simulink model "rule_DJ"  (R2021a)
settings: Solver=FixedStepAuto  StartTime=0.0  StopTime=8.9  FixedStep=1/30  RelTol=1e-3
values from neighbouring files (symbols this model uses):
  y = zeros(10,4)    [simulate.m]
libraries: simulink x17
(part 2 of 3)

== matlab function rule_DJ/EnabledSubsystem/EnabledSubsystem/changeright ==
  data: Egolane input; initial_lane input; Ego input; y1 output; y_line input; maxt_changeline output; staticinfo input; cmplt_change output
function [y1,maxt_changeline,cmplt_change] = fcn(Egolane,initial_lane,Ego,y_line,staticinfo)
%%参数注释
%{
sEgo = 0;                  %自车纵坐标（始终为零）(m)
dEgo = Ego(2);             %自车横坐标(m)
vxEgo = Ego(3);            %自车纵向速度(m/s)
vyEgo = Ego(4);            %自车横向速度(m/s)
phiEgo = Ego(5);           %自车航向角（相对路径切向夹角，逆时针为正） (rad)
laneEgo = Ego(6);          %自车所在车道
wEgo = Ego(7);             %自车横向宽度(m)
aEgo = Ego(8);             %自车质心到最前端的距离(m)
bEgo = Ego(9);             %自车质心到最前端的距离(m)
sTgt_ot = Tgt_ot(1);       %超车目标纵坐标(m)
dTgt_ot = Tgt_ot(2);       %超车目标横坐标(m)
vxTgt_ot = Tgt_ot(3);      %超车目标纵向速度(m/s)
vyTgt_ot = Tgt_ot(4);      %超车目标横向速度(m/s)
sTgt_f = Tgt_f(1);         %前车纵坐标(m)
dTgt_f = Tgt_f(2);         %前车横坐标(m)
vxTgt_f = Tgt_f(3);        %前车纵向速度(m/s)
vyTgt_f = Tgt_f(4);        %前车横向速度(m/s)
sTgt_lf = Tgt_lf(1);       %左前车纵坐标(m)
dTgt_lf = Tgt_lf(2);       %左前车横坐标(m)
vxTgt_lf = Tgt_lf(3);      %左前车纵向速度(m/s)
vyTgt_lf = Tgt_lf(4);      %左前车横向速度(m/s)
Tgt_lr, Tgt_rf, Tgt_rr与左前车类似，分别表示相对自车的左后车辆，右前车辆以及右后车辆
dlaneline =[dlaneline-1,dlaneline-2,……]
%同向车道内车道线横向坐标集，最靠近道路中心线的一侧为-1，往外依次递减
TTCx_f = Threshold_para(1);             %纵向安全距离
TTCx_lr = Threshold_para(2);            %超车道后方安全距离
TTCx_lf = Threshold_para(3);            %超车道前方安全距离
t_chngln = Threshold_para(4);           %换道持续最大时间
overtake_deltav = Threshold_para(5);    %超车速度差
sf_dist_return = Threshold_para(6);     %返回原车道与后方车辆的安全，由于超车时自车速度应大于被超车辆
TTCx_rf = Threshold_para(7);            %原车道前方安全距离
%}
%%

%参数需求
Egox = Ego.EgoX;
Egoy = Ego.EgoY;                    %自车y坐标(m)
Egovx = Ego.EgoVx;
Egovy = Ego.EgoVy;
Egol = Ego.Length;
Egow = Ego.Width;
Egotheta = Ego.EgoTheta;
laneEgo = Egolane;          %自车所在车道
maxt_changeline = staticinfo(6);


%计算向左换道所用时间
lf_Ego = Egoy + 0.5 * Egol * sin(Egotheta) - 0.5 * Egow * cos(Egotheta); %左前角车辆横坐标
rf_Ego = Egoy + 0.5 * Egol * sin(Egotheta) + 0.5 * Egow * cos(Egotheta); %右前角车辆横坐标
lr_Ego = Egoy - 0.5 * Egol * sin(Egotheta) - 0.5 * Egow * cos(Egotheta); %左前角车辆横坐标
rr_Ego = Egoy - 0.5 * Egol * sin(Egotheta) + 0.5 * Egow * cos(Egotheta); %右后角车辆横坐标
if Egovx > 0 && Egovy > 0
    changeleft = 1;
    Egoxf_line = polyval(y_line(initial_lane,:),Egox+0.5*Egol*cos(Egotheta));
    changeright = sign((rf_Ego-Egoxf_line) * (lr_Ego-Egoxf_line));
elseif Egovx > 0 && Egovy < 0
    Egoxf_line = polyval(y_line(initial_lane+1,:),Egox+0.5*Egol*cos(Egotheta));
    changeleft = sign((lf_Ego-Egoxf_line) * (rr_Ego-Egoxf_line));
    changeright = 1;
elseif Egovx < 0 && Egovy > 0
    Egoxf_line = polyval(y_line(initial_lane,:),Egox+0.5*Egol*cos(Egotheta));
    changeleft = sign((lf_Ego-Egoxf_line) * (rr_Ego-Egoxf_line));
    changeright = 1;
else
    changeleft = 1;
    Egoxf_line = polyval(y_line(initial_lane+1,:),Egox+0.5*Egol*cos(Egotheta));
    changeright = sign((rf_Ego-Egoxf_line) * (lr_Ego-Egoxf_line));
end

if changeright <= 0
    y1 = true;       %y1为true的时间即为换道时间，该时间不得超过10s
else
    y1 = false;
end

if laneEgo == initial_lane && changeleft > 0 && changeright > 0
    cmplt_change = 1;
elseif laneEgo ~= initial_lane && changeleft > 0 && changeright > 0
    cmplt_change = 2;
elseif laneEgo ~= initial_lane && changeright <= 0
    cmplt_change = 3;
else
    cmplt_change = 0;
end

end

== matlab function rule_DJ/trigger_rule78 ==
  data: y_line input; y output; Egolaneid input
function y = fcn(y_line,Egolaneid)
%%

%参数需求
lane_type = Egolaneid;

%高速主路限速触发条件判断
if lane_type ~= 1 && lane_type ~= size(y_line,1)-1        %自车所属车道类型为主干道则条件有效
    y = 1;
else
    y = 0;
end

== matlab function rule_DJ/EnabledSubsystem/EnabledSubsystem/distance/zoning ==
  data: Ego input; Tgt_f output; Tgt input; y_line input; Tgt_b output; Tgt_lf output; Tgt_lr output; Tgt_rf output; Tgt_rr output; Egolane output
function [Tgt_f,Tgt_b,Tgt_lf,Tgt_lr,Tgt_rf,Tgt_rr,Egolane] = fcn(Ego,Tgt,y_line)
%{
根据HighD数据集提供的信息，通过确定自车所在的位置，以及他车的坐标，判断他车相对于自车的方位
%}
Egox = Ego.EgoX;
Egoy = Ego.EgoY;
Egovx = Ego.EgoVx;
Tgtx = Tgt.TgtX;
Tgty = Tgt.TgtY;
Tgtvx = Tgt.TgtVx;
Tgtl = Tgt.Length;
Tgtw = Tgt.Width;

%%判断自车所在的车道
for i = 1:size(y_line,1)
    if Egoy >= polyval(y_line(i,:),Egox);
        Egolane = i-1;
        break
    else
        Egolane = i;
    end
end

%%对周围的他车进行方位分割
if Egolane<size(y_line,1)/2  %说明自车在地图中为向右行驶（下方）车辆
    Flag1 = Tgtx > Egox;      %他车位于自车之前
    Flag2 = Tgtx <= Egox;     %他车位于自车之后
    if Egolane == 1                                   %自车位于车道1
        Flag3 = (Tgty>=polyval(y_line(2,:),Tgtx) & Tgty<polyval(y_line(1,:),Tgtx));      %同车道他车
        Flag5 = (Tgty>=polyval(y_line(3,:),Tgtx) & Tgty<polyval(y_line(2,:),Tgtx));;      %左侧车道他车
        [m, n] = size(Flag3);
        Flag4 = false(m,n);%右侧车道他车
    elseif Egolane>1 && Egolane<size(y_line,1)/2           %自车位于车道中间车道
        Flag3 = (Tgty>=polyval(y_line(Egolane+1,:),Tgtx) & Tgty<polyval(y_line(Egolane,:),Tgtx));   %同车道他车
        Flag5 = (Tgty>=polyval(y_line(Egolane+2,:),Tgtx) & Tgty<polyval(y_line(Egolane+1,:),Tgtx)); %左侧车道他车
        Flag4 = (Tgty>=polyval(y_line(Egolane,:),Tgtx) & Tgty<polyval(y_line(Egolane-1,:),Tgtx));   %右侧车道他车
    else                                                  %自车位于车道3
        Flag3 = (Tgty>=polyval(y_line(Egolane+1,:),Tgtx) & Tgty<polyval(y_line(Egolane,:),Tgtx));  %同车道他车
        [m, n] = size(Flag3);
        Flag5 = false(m,n);
        Flag4 = (Tgty>=polyval(y_line(Egolane,:),Tgtx) & Tgty<polyval(y_line(Egolane-1,:),Tgtx));  %右侧车道他车
    end
else
    Flag1 = Tgtx <= Egox;    %他车位于自车之前
    Flag2 = Tgtx > Egox;     %他车位于自车之后
    if Egolane == size(y_line,1)/2+1                                   %自车位于车道6
        Flag3 = (Tgty>=polyval(y_line(Egolane+1,:),Tgtx) & Tgty<polyval(y_line(Egolane,:),Tgtx));  %同车道他车
        Flag4 = (Tgty>=polyval(y_line(Egolane+2,:),Tgtx) & Tgty<polyval(y_line(Egolane+1,:),Tgtx));  %右侧车道他车
        [m, n] = size(Flag3);
        Flag5 = false(m,n);
    elseif Egolane>size(y_line,1)/2+1 && Egolane<=size(y_line,1)-2           %自车位于车道-2
        Flag3 = (Tgty>=polyval(y_line(Egolane+1,:),Tgtx) & Tgty<polyval(y_line(Egolane,:),Tgtx));  %同车道他车
        Flag4 = (Tgty>=polyval(y_line(Egolane+2,:),Tgtx) & Tgty<polyval(y_line(Egolane+1,:),Tgtx));  %右侧车道他车
        Flag5 = (Tgty>=polyval(y_line(Egolane,:),Tgtx) & Tgty<polyval(y_line(Egolane-1,:),Tgtx));  %左侧车道他车
    else                                                  %自车位于车道-3
        Flag3 = (Tgty>=polyval(y_line(Egolane+1,:),Tgtx) & Tgty<polyval(y_line(Egolane,:),Tgtx));               %同车道他车
        [m, n] = size(Flag3);
        Flag4 = false(m,n);
        Flag5 = (Tgty>=polyval(y_line(Egolane,:),Tgtx) & Tgty<polyval(y_line(Egolane+1,:),Tgtx)); %左侧车道他车
    end
end

%%筛选六个方位中离自车最近的车，即每个方位区域只保留一辆车
Flag_f = Flag1 & Flag3;      %同车道前车
if any(Flag_f)
    f_min = min(abs(Tgtx(Flag_f) - Egox));
    Tgtx_f = (sign(min(Tgtx(Flag_f) - Egox)) * f_min) + Egox;
    [col_f,~] = find(abs(Tgtx-Tgtx_f)<=0.0001 & Flag_f == true);
    if ~isempty(col_f)
        Tgty_f = Tgty(col_f(1));
        Tgtvx_f = Tgtvx(col_f(1));
        Tgtl_f = Tgtl(col_f(1));
        Tgtw_f = Tgtw(col_f(1));
    else
        Tgty_f = 0;
        Tgtvx_f = 0;
        Tgtl_f = 0;
        Tgtw_f = 0;
    end
else
    f_min = 0;
    Tgtx_f = 2000;
    Tgty_f = 2000;
    Tgtvx_f = 2000;
    Tgtl_f = 2000;
    Tgtw_f = 2000;
end
Tgt_f = [Tgtx_f, Tgty_f, Tgtvx_f, Tgtl_f, Tgtw_f];
Flag_b = Flag2 & Flag3;      %同车道后车
if any(Flag_b)
    b_min = min(abs(Tgtx(Flag_b) - Egox));
    Tgtx_b = (sign(min(Tgtx(Flag_b) - Egox)) * b_min) + Egox;
    [col_b,~] = find(abs(Tgtx-Tgtx_b)<=0.0001 & Flag_b == true);
    if ~isempty(col_b)
        Tgty_b = Tgty(col_b(1));
        Tgtvx_b = Tgtvx(col_b(1));
        Tgtl_b = Tgtl(col_b(1));
        Tgtw_b = Tgtw(col_b(1));
    else
        Tgty_b = 0;
        Tgtvx_b = 0;
        Tgtl_b = 0;
        Tgtw_b = 0;
    end
else
    b_min = 0;
    Tgtx_b = 2000;
    Tgty_b = 2000;
    Tgtvx_b = 2000;
    Tgtl_b = 2000;
    Tgtw_b = 2000;
end
Tgt_b = [Tgtx_b, Tgty_b, Tgtvx_b, Tgtl_b, Tgtw_b];
Flag_lf = (Flag1 & Flag5);     %左侧车道前车
if any(Flag_lf)
    lf_min = min(abs(Tgtx(Flag_lf) - Egox));
    Tgtx_lf = (sign(min(Tgtx(Flag_lf) - Egox)) * lf_min) + Egox;
    [col_lf,~] = find(abs(Tgtx-Tgtx_lf)<=0.0001 & Flag_lf == true);
    if ~isempty(col_lf)
        Tgty_lf = Tgty(col_lf(1));
        Tgtvx_lf = Tgtvx(col_lf(1));
        Tgtl_lf = Tgtl(col_lf(1));
        Tgtw_lf = Tgtw(col_lf(1));
    else
        Tgty_lf = 0;
        Tgtvx_lf = 0;
        Tgtl_lf = 0;
        Tgtw_lf = 0;
    end
else
    lf_min = 0;
    Tgtx_lf = 2000;
    Tgty_lf = 2000;
    Tgtvx_lf = 2000;
    Tgtl_lf = 2000;
    Tgtw_lf = 2000;
end
Tgt_lf = [Tgtx_lf, Tgty_lf, Tgtvx_lf, Tgtl_lf, Tgtw_lf];
Flag_lr = Flag2 & Flag5;     %左侧车道后车
if any(Flag_lr)
    lr_min = min(abs(Tgtx(Flag_lr) - Egox));
    Tgtx_lr = (sign(min(Tgtx(Flag_lr) - Egox)) * lr_min) + Egox;
    [col_lr,~] = find(abs(Tgtx-Tgtx_lr)<=0.0001 & Flag_lr == true);
    if ~isempty(col_lr)
        Tgty_lr = Tgty(col_lr(1));
        Tgtvx_lr = Tgtvx(col_lr(1));
        Tgtl_lr = Tgtl(col_lr(1));
        Tgtw_lr = Tgtw(col_lr(1));
    else
        Tgty_lr = 0;
        Tgtvx_lr = 0;
        Tgtl_lr = 0;
        Tgtw_lr = 0;
    end
else
    lr_min = 0;
    Tgtx_lr= 2000;
    Tgty_lr = 2000;
    Tgtvx_lr = 2000;
    Tgtl_lr = 2000;
    Tgtw_lr = 2000;
end
Tgt_lr = [Tgtx_lr, Tgty_lr, Tgtvx_lr, Tgtl_lr, Tgtw_lr];
Flag_rf = Flag1 & Flag4;     %右侧车道前车
if any(Flag_rf)
    rf_min = min(abs(Tgtx(Flag_rf) - Egox));
    Tgtx_rf = (sign(min(Tgtx(Flag_rf) - Egox)) * rf_min) + Egox;
    [col_rf,~] = find(abs(Tgtx-Tgtx_rf)<=0.0001 & Flag_rf == true);
    if ~isempty(col_rf)
        Tgty_rf = Tgty(col_rf(1));
        Tgtvx_rf = Tgtvx(col_rf(1));
        Tgtl_rf = Tgtl(col_rf(1));
        Tgtw_rf = Tgtw(col_rf(1));
    else
        Tgty_rf = 0;
        Tgtvx_rf = 0;
        Tgtl_rf = 0;
        Tgtw_rf = 0;
    end
else
    rf_min = 0;
    Tgtx_rf = 2000;
    Tgty_rf = 2000;
    Tgtvx_rf = 2000;
    Tgtl_rf = 2000;
    Tgtw_rf = 2000;
end
Tgt_rf = [Tgtx_rf, Tgty_rf, Tgtvx_rf, Tgtl_rf, Tgtw_rf];
Flag_rr = Flag2 & Flag4;     %同车道后车
if any(Flag_rr)
    rr_min = min(abs(Tgtx(Flag_rr) - Egox));
    Tgtx_rr = (sign(min(Tgtx(Flag_rr) - Egox)) * rr_min) + Egox;
    [col_rr,~] = find(abs(Tgtx-Tgtx_rr)<=0.0001 & Flag_rr == true);
    if ~isempty(col_rr)
        Tgty_rr = Tgty(col_rr(1));
        Tgtvx_rr = Tgtvx(col_rr(1));
        Tgtl_rr = Tgtl(col_rr(1));
        Tgtw_rr = Tgtw(col_rr(1));
    else
        Tgty_rr = 0;
        Tgtvx_rr = 0;
        Tgtl_rr = 0;
        Tgtw_rr = 0;
    end
else
    rr_min = 0;
    Tgtx_rr = 2000;
    Tgty_rr = 2000;
    Tgtvx_rr = 2000;
    Tgtl_rr = 2000;
    Tgtw_rr = 2000;
end
Tgt_rr = [Tgtx_rr, Tgty_rr, Tgtvx_rr, Tgtl_rr, Tgtw_rr];

== matlab function rule_DJ/EnabledSubsystem/changelane ==
  data: initial_lane input; Egolane input; Ego input; y1 output; maxt_changeline output; y_line input; cmplt_change output; staticinfo input
function [y1,maxt_changeline,cmplt_change] = fcn(initial_lane,Egolane,Ego,y_line,staticinfo)
%%参数注释
%{
sEgo = 0;                  %自车纵坐标（始终为零）(m)
dEgo = Ego(2);             %自车横坐标(m)
vxEgo = Ego(3);            %自车纵向速度(m/s)
vyEgo = Ego(4);            %自车横向速度(m/s)
phiEgo = Ego(5);           %自车航向角（相对路径切向夹角，逆时针为正） (rad)
laneEgo = Ego(6);          %自车所在车道
wEgo = Ego(7);             %自车横向宽度(m)
aEgo = Ego(8);             %自车质心到最前端的距离(m)
bEgo = Ego(9);             %自车质心到最前端的距离(m)
sTgt_ot = Tgt_ot(1);       %超车目标纵坐标(m)
dTgt_ot = Tgt_ot(2);       %超车目标横坐标(m)
vxTgt_ot = Tgt_ot(3);      %超车目标纵向速度(m/s)
vyTgt_ot = Tgt_ot(4);      %超车目标横向速度(m/s)
sTgt_f = Tgt_f(1);         %前车纵坐标(m)
dTgt_f = Tgt_f(2);         %前车横坐标(m)
vxTgt_f = Tgt_f(3);        %前车纵向速度(m/s)
vyTgt_f = Tgt_f(4);        %前车横向速度(m/s)
sTgt_lf = Tgt_lf(1);       %左前车纵坐标(m)
dTgt_lf = Tgt_lf(2);       %左前车横坐标(m)
vxTgt_lf = Tgt_lf(3);      %左前车纵向速度(m/s)
vyTgt_lf = Tgt_lf(4);      %左前车横向速度(m/s)
Tgt_lr, Tgt_rf, Tgt_rr与左前车类似，分别表示相对自车的左后车辆，右前车辆以及右后车辆
dlaneline =[dlaneline-1,dlaneline-2,……]
%同向车道内车道线横向坐标集，最靠近道路中心线的一侧为-1，往外依次递减
TTCx_f = Threshold_para(1);             %纵向安全距离
TTCx_lr = Threshold_para(2);            %超车道后方安全距离
TTCx_lf = Threshold_para(3);            %超车道前方安全距离
t_chngln = Threshold_para(4);           %换道持续最大时间
overtake_deltav = Threshold_para(5);    %超车速度差
sf_dist_return = Threshold_para(6);     %返回原车道与后方车辆的安全，由于超车时自车速度应大于被超车辆
TTCx_rf = Threshold_para(7);            %原车道前方安全距离
%}
%%

%参数需求
Egox = Ego.EgoX;
Egoy = Ego.EgoY;                    %自车y坐标(m)
Egovx = Ego.EgoVx;
Egovy = Ego.EgoVy;
Egol = Ego.Length;
Egow = Ego.Width;
laneEgo = Egolane;
maxt_changeline = staticinfo(6);
if Egovx >0
    Egotheta = 0;
else
    Egotheta = pi;
end
%计算向左换道所用时间
lf_Ego = Egoy + 0.5 * Egol * sin(Egotheta) - 0.5 * Egow * cos(Egotheta); %左前角车辆横坐标
rf_Ego = Egoy + 0.5 * Egol * sin(Egotheta) + 0.5 * Egow * cos(Egotheta); %右前角车辆横坐标
lr_Ego = Egoy - 0.5 * Egol * sin(Egotheta) - 0.5 * Egow * cos(Egotheta); %左前角车辆横坐标
rr_Ego = Egoy - 0.5 * Egol * sin(Egotheta) + 0.5 * Egow * cos(Egotheta); %右后角车辆横坐标

if Egovx > 0 && Egovy > 0
    changeleft = 1;
    Egoxf_line = polyval(y_line(initial_lane,:),Egox+0.5*Egol*cos(Egotheta));
    changeright = sign((rf_Ego-Egoxf_line) * (lr_Ego-Egoxf_line));
elseif Egovx > 0 && Egovy < 0
    Egoxf_line = polyval(y_line(initial_lane+1,:),Egox+0.5*Egol*cos(Egotheta));
    changeleft = sign((lf_Ego-Egoxf_line) * (rr_Ego-Egoxf_line));
    changeright = 1;
elseif Egovx < 0 && Egovy > 0
    Egoxf_line = polyval(y_line(initial_lane,:),Egox+0.5*Egol*cos(Egotheta));
    changeleft = sign((lf_Ego-Egoxf_line) * (rr_Ego-Egoxf_line));
    changeright = 1;
else
    changeleft = 1;
    Egoxf_line = polyval(y_line(initial_lane+1,:),Egox+0.5*Egol*cos(Egotheta));
    changeright = sign((rf_Ego-Egoxf_line) * (lr_Ego-Egoxf_line));
end

if changeleft <= 0
    y1 = true;       %y1为true的时间即为换道时间，该时间不得超过10s
else
    y1 = false;
end

if Egovx > 0
    if laneEgo == initial_lane+1 && changeleft > 0 && changeright > 0
        cmplt_change = 1;
    elseif laneEgo == initial_lane && changeleft > 0 && changeright > 0
        cmplt_change = 2;
    elseif laneEgo == initial_lane-1 && changeleft > 0 && changeright > 0
        cmplt_change = 3;
    elseif laneEgo == initial_lane && changeleft <= 0
        cmplt_change = 4;
    else 
        cmplt_change = 0;
    end
else
    if laneEgo == initial_lane-1 && changeleft > 0 && changeright > 0
        cmplt_change = 1;
    elseif laneEgo == initial_lane && changeleft > 0 && changeright > 0
        cmplt_change = 2;
    elseif laneEgo == initial_lane+1 && changeleft > 0 && changeright > 0
        cmplt_change = 3;
    elseif laneEgo == initial_lane && changeleft <= 0
        cmplt_change = 4;
    else 
        cmplt_change = 0;
    end
end

end

== matlab function rule_DJ/EnabledSubsystem/distance/zoning ==
  data: Ego input; Tgt_f output; Tgt input; y_line input; Tgt_b output; Tgt_lf output; Tgt_lr output; Tgt_rf output; Tgt_rr output; Egolane output
function [Tgt_f,Tgt_b,Tgt_lf,Tgt_lr,Tgt_rf,Tgt_rr,Egolane] = fcn(Ego,Tgt,y_line)
%{
根据HighD数据集提供的信息，通过确定自车所在的位置，以及他车的坐标，判断他车相对于自车的方位
%}
Egox = Ego.EgoX;
Egoy = Ego.EgoY;
Egovx = Ego.EgoVx;
Tgtx = Tgt.TgtX;
Tgty = Tgt.TgtY;
Tgtvx = Tgt.TgtVx;
Tgtl = Tgt.Length;
Tgtw = Tgt.Width;

%%判断自车所在的车道
for i = 1:size(y_line,1)
    if Egoy >= polyval(y_line(i,:),Egox);
        Egolane = i-1;
        break
    else
        Egolane = i;
    end
end

%%对周围的他车进行方位分割
if Egolane<size(y_line,1)/2  %说明自车在地图中为向右行驶（下方）车辆
    Flag1 = Tgtx > Egox;      %他车位于自车之前
    Flag2 = Tgtx <= Egox;     %他车位于自车之后
    if Egolane == 1                                   %自车位于车道1
        Flag3 = (Tgty>=polyval(y_line(2,:),Tgtx) & Tgty<polyval(y_line(1,:),Tgtx));      %同车道他车
        Flag5 = (Tgty>=polyval(y_line(3,:),Tgtx) & Tgty<polyval(y_line(2,:),Tgtx));;      %左侧车道他车
        [m, n] = size(Flag3);
        Flag4 = false(m,n);%右侧车道他车
    elseif Egolane>1 && Egolane<size(y_line,1)/2           %自车位于车道中间车道
        Flag3 = (Tgty>=polyval(y_line(Egolane+1,:),Tgtx) & Tgty<polyval(y_line(Egolane,:),Tgtx));   %同车道他车
        Flag5 = (Tgty>=polyval(y_line(Egolane+2,:),Tgtx) & Tgty<polyval(y_line(Egolane+1,:),Tgtx)); %左侧车道他车
        Flag4 = (Tgty>=polyval(y_line(Egolane,:),Tgtx) & Tgty<polyval(y_line(Egolane-1,:),Tgtx));   %右侧车道他车
    else                                                  %自车位于车道3
        Flag3 = (Tgty>=polyval(y_line(Egolane+1,:),Tgtx) & Tgty<polyval(y_line(Egolane,:),Tgtx));  %同车道他车
        [m, n] = size(Flag3);
        Flag5 = false(m,n);
        Flag4 = (Tgty>=polyval(y_line(Egolane,:),Tgtx) & Tgty<polyval(y_line(Egolane-1,:),Tgtx));  %右侧车道他车
    end
else
    Flag1 = Tgtx <= Egox;    %他车位于自车之前
    Flag2 = Tgtx > Egox;     %他车位于自车之后
    if Egolane == size(y_line,1)/2+1                                   %自车位于车道6
        Flag3 = (Tgty>=polyval(y_line(Egolane+1,:),Tgtx) & Tgty<polyval(y_line(Egolane,:),Tgtx));  %同车道他车
        Flag4 = (Tgty>=polyval(y_line(Egolane+2,:),Tgtx) & Tgty<polyval(y_line(Egolane+1,:),Tgtx));  %右侧车道他车
        [m, n] = size(Flag3);
        Flag5 = false(m,n);
    elseif Egolane>size(y_line,1)/2+1 && Egolane<=size(y_line,1)-2           %自车位于车道-2
        Flag3 = (Tgty>=polyval(y_line(Egolane+1,:),Tgtx) & Tgty<polyval(y_line(Egolane,:),Tgtx));  %同车道他车
        Flag4 = (Tgty>=polyval(y_line(Egolane+2,:),Tgtx) & Tgty<polyval(y_line(Egolane+1,:),Tgtx));  %右侧车道他车
        Flag5 = (Tgty>=polyval(y_line(Egolane,:),Tgtx) & Tgty<polyval(y_line(Egolane-1,:),Tgtx));  %左侧车道他车
    else                                                  %自车位于车道-3
        Flag3 = (Tgty>=polyval(y_line(Egolane+1,:),Tgtx) & Tgty<polyval(y_line(Egolane,:),Tgtx));               %同车道他车
        [m, n] = size(Flag3);
        Flag4 = false(m,n);
        Flag5 = (Tgty>=polyval(y_line(Egolane,:),Tgtx) & Tgty<polyval(y_line(Egolane+1,:),Tgtx)); %左侧车道他车
    end
end

%%筛选六个方位中离自车最近的车，即每个方位区域只保留一辆车
Flag_f = Flag1 & Flag3;      %同车道前车
if any(Flag_f)
    f_min = min(abs(Tgtx(Flag_f) - Egox));
    Tgtx_f = (sign(min(Tgtx(Flag_f) - Egox)) * f_min) + Egox;
    [col_f,~] = find(abs(Tgtx-Tgtx_f)<=0.0001 & Flag_f == true);
    if ~isempty(col_f)
        Tgty_f = Tgty(col_f(1));
        Tgtvx_f = Tgtvx(col_f(1));
        Tgtl_f = Tgtl(col_f(1));
        Tgtw_f = Tgtw(col_f(1));
    else
        Tgty_f = 0;
        Tgtvx_f = 0;
        Tgtl_f = 0;
        Tgtw_f = 0;
    end
else
    f_min = 0;
    Tgtx_f = 2000;
    Tgty_f = 2000;
    Tgtvx_f = 2000;
    Tgtl_f = 2000;
    Tgtw_f = 2000;
end
Tgt_f = [Tgtx_f, Tgty_f, Tgtvx_f, Tgtl_f, Tgtw_f];
Flag_b = Flag2 & Flag3;      %同车道后车
if any(Flag_b)
    b_min = min(abs(Tgtx(Flag_b) - Egox));
    Tgtx_b = (sign(min(Tgtx(Flag_b) - Egox)) * b_min) + Egox;
    [col_b,~] = find(abs(Tgtx-Tgtx_b)<=0.0001 & Flag_b == true);
    if ~isempty(col_b)
        Tgty_b = Tgty(col_b(1));
        Tgtvx_b = Tgtvx(col_b(1));
        Tgtl_b = Tgtl(col_b(1));
        Tgtw_b = Tgtw(col_b(1));
    else
        Tgty_b = 0;
        Tgtvx_b = 0;
        Tgtl_b = 0;
        Tgtw_b = 0;
    end
else
    b_min = 0;
    Tgtx_b = 2000;
    Tgty_b = 2000;
    Tgtvx_b = 2000;
    Tgtl_b = 2000;
    Tgtw_b = 2000;
end
Tgt_b = [Tgtx_b, Tgty_b, Tgtvx_b, Tgtl_b, Tgtw_b];
Flag_lf = (Flag1 & Flag5);     %左侧车道前车
if any(Flag_lf)
    lf_min = min(abs(Tgtx(Flag_lf) - Egox));
    Tgtx_lf = (sign(min(Tgtx(Flag_lf) - Egox)) * lf_min) + Egox;
    [col_lf,~] = find(abs(Tgtx-Tgtx_lf)<=0.0001 & Flag_lf == true);
    if ~isempty(col_lf)
        Tgty_lf = Tgty(col_lf(1));
        Tgtvx_lf = Tgtvx(col_lf(1));
        Tgtl_lf = Tgtl(col_lf(1));
        Tgtw_lf = Tgtw(col_lf(1));
    else
        Tgty_lf = 0;
        Tgtvx_lf = 0;
        Tgtl_lf = 0;
        Tgtw_lf = 0;
    end
else
    lf_min = 0;
    Tgtx_lf = 2000;
    Tgty_lf = 2000;
    Tgtvx_lf = 2000;
    Tgtl_lf = 2000;
    Tgtw_lf = 2000;
end
Tgt_lf = [Tgtx_lf, Tgty_lf, Tgtvx_lf, Tgtl_lf, Tgtw_lf];
Flag_lr = Flag2 & Flag5;     %左侧车道后车
if any(Flag_lr)
    lr_min = min(abs(Tgtx(Flag_lr) - Egox));
    Tgtx_lr = (sign(min(Tgtx(Flag_lr) - Egox)) * lr_min) + Egox;
    [col_lr,~] = find(abs(Tgtx-Tgtx_lr)<=0.0001 & Flag_lr == true);
    if ~isempty(col_lr)
        Tgty_lr = Tgty(col_lr(1));
        Tgtvx_lr = Tgtvx(col_lr(1));
        Tgtl_lr = Tgtl(col_lr(1));
        Tgtw_lr = Tgtw(col_lr(1));
    else
        Tgty_lr = 0;
        Tgtvx_lr = 0;
        Tgtl_lr = 0;
        Tgtw_lr = 0;
    end
else
    lr_min = 0;
    Tgtx_lr= 2000;
    Tgty_lr = 2000;
    Tgtvx_lr = 2000;
    Tgtl_lr = 2000;
    Tgtw_lr = 2000;
end
Tgt_lr = [Tgtx_lr, Tgty_lr, Tgtvx_lr, Tgtl_lr, Tgtw_lr];
Flag_rf = Flag1 & Flag4;     %右侧车道前车
if any(Flag_rf)
    rf_min = min(abs(Tgtx(Flag_rf) - Egox));
    Tgtx_rf = (sign(min(Tgtx(Flag_rf) - Egox)) * rf_min) + Egox;
    [col_rf,~] = find(abs(Tgtx-Tgtx_rf)<=0.0001 & Flag_rf == true);
    if ~isempty(col_rf)
        Tgty_rf = Tgty(col_rf(1));
        Tgtvx_rf = Tgtvx(col_rf(1));
        Tgtl_rf = Tgtl(col_rf(1));
        Tgtw_rf = Tgtw(col_rf(1));
    else
        Tgty_rf = 0;
        Tgtvx_rf = 0;
        Tgtl_rf = 0;
        Tgtw_rf = 0;
    end
else
    rf_min = 0;
    Tgtx_rf = 2000;
    Tgty_rf = 2000;
    Tgtvx_rf = 2000;
    Tgtl_rf = 2000;
    Tgtw_rf = 2000;
end
Tgt_rf = [Tgtx_rf, Tgty_rf, Tgtvx_rf, Tgtl_rf, Tgtw_rf];
Flag_rr = Flag2 & Flag4;     %同车道后车
if any(Flag_rr)
    rr_min = min(abs(Tgtx(Flag_rr) - Egox));
    Tgtx_rr = (sign(min(Tgtx(Flag_rr) - Egox)) * rr_min) + Egox;
    [col_rr,~] = find(abs(Tgtx-Tgtx_rr)<=0.0001 & Flag_rr == true);
    if ~isempty(col_rr)
        Tgty_rr = Tgty(col_rr(1));
        Tgtvx_rr = Tgtvx(col_rr(1));
        Tgtl_rr = Tgtl(col_rr(1));
        Tgtw_rr = Tgtw(col_rr(1));
    else
        Tgty_rr = 0;
        Tgtvx_rr = 0;
        Tgtl_rr = 0;
        Tgtw_rr = 0;
    end
else
    rr_min = 0;
    Tgtx_rr = 2000;
    Tgty_rr = 2000;
    Tgtvx_rr = 2000;
    Tgtl_rr = 2000;
    Tgtw_rr = 2000;
end
Tgt_rr = [Tgtx_rr, Tgty_rr, Tgtvx_rr, Tgtl_rr, Tgtw_rr];

== matlab function rule_DJ/EnabledSubsystem/distance/beforeovertaking ==
  data: y1 output; y2 output; y3 output; Ego input; Tgt_f input; Tgt_lf input; Tgt_lr input; Threshold_para input
function [y1,y2,y3] = fcn(Ego,Tgt_f,Tgt_lf,Tgt_lr,Threshold_para)
%%参数注释
%{
sEgo = 0;                  %自车纵坐标（始终为零）(m)
dEgo = Ego(2);             %自车横坐标(m)
vxEgo = Ego(3);            %自车纵向速度(m/s)
vyEgo = Ego(4);            %自车横向速度(m/s)
phiEgo = Ego(5);           %自车航向角（相对路径切向夹角，逆时针为正） (rad)
laneEgo = Ego(6);          %自车所在车道
wEgo = Ego(6);             %自车横向宽度(m)
aEgo = Ego(7);             %自车质心到最前端的距离(m)
bEgo = Ego(8);             %自车质心到最前端的距离(m)
sTgt_ot = Tgt_ot(1);         %超车目标纵坐标(m)
dTgt_ot = Tgt_ot(2);         %超车目标横坐标(m)
vxTgt_ot = Tgt_ot(3);        %超车目标纵向速度(m/s)
vyTgt_ot = Tgt_ot(4);        %超车目标横向速度(m/s)
sTgt_f = Tgt_f(1);         %前车纵坐标(m)
dTgt_f = Tgt_f(2);         %前车横坐标(m)
vxTgt_f = Tgt_f(3);        %前车纵向速度(m/s)
vyTgt_f = Tgt_f(4);        %前车横向速度(m/s)
sTgt_lf = Tgt_lf(1);       %左前车纵坐标(m)
dTgt_lf = Tgt_lf(2);       %左前车横坐标(m)
vxTgt_lf = Tgt_lf(3);      %左前车纵向速度(m/s)
vyTgt_lf = Tgt_lf(4);      %左前车横向速度(m/s)
Tgt_lr, Tgt_rf, Tgt_rr与左前车类似，分别表示相对自车的左后车辆，右前车辆以及右后车辆
dlaneline =[dlaneline-1,dlaneline-2,……]
%同向车道内车道线横向坐标集，最靠近道路中心线的一侧为-1，往外依次递减
TTCx_f = Threshold_para(1);             %纵向安全距离
TTCx_lr = Threshold_para(2);            %超车道后方安全距离
TTCx_lf = Threshold_para(3);            %超车道前方安全距离
t_chngln = Threshold_para(4);           %换道持续最大时间
overtake_deltav = Threshold_para(5);    %超车速度差
sf_dist_return = Threshold_para(6);     %返回原车道与后方车辆的安全，由于超车时自车速度应大于被超车辆
TTCx_rf = Threshold_para(7);            %原车道前方安全距离
%}
%%

%参数需求

Tgtx_lr = Tgt_lr(1);              %frenet坐标系下左侧车道后方车辆坐标
Tgty_lr = Tgt_lr(2);              
Tgtvx_lr = Tgt_lr(3);             %左前车纵向速度(m/s)
Egox = Ego.EgoX;                    %自车纵坐标（）
Egovx = Ego.EgoVx;                  %自车纵向速度(m/s)
Tgtx_f = Tgt_f(1);              %超车目标纵坐标(m)
Tgtvx_f = Tgt_f(3);             %超车目标纵向速度(m/s)
Tgtx_lf = Tgt_lf(1);              %frenet坐标系下左侧车道前方车辆坐标
Tgty_lf = Tgt_lf(2);
Tgtvx_lf = Tgt_lf(3);             %左前车纵向速度(m/s)
TTCx = Threshold_para(7);      %超车道后方安全距离

%与前车的安全距离判断
if abs(Tgtx_f-Egox) >= abs(Egovx - Tgtvx_f) * TTCx
    y1 = 0;
else
    y1 = 1;
end
%与左前车的安全距离判断
if Tgtx_lf ~= 2000 && Tgty_lf ~= 2000 && abs(Egovx)>abs(Tgtvx_lf)    %坐标不为0视为存在左前车
    if abs(Tgtx_lf-Egox) >= abs(Egovx - Tgtvx_lf) * TTCx 
        y2 = 0;
    else
        y2 = 1;
    end
else
    y2 = 0;
end
%与左后车的安全距离判断
if Tgtx_lr ~= 2000 && Tgty_lr ~= 2000 && abs(Egovx)<abs(Tgtvx_lr)    %坐标不为0视为存在左后车
    if abs(Tgtx_lr-Egox) >= abs(Egovx - Tgtvx_lr) * TTCx 
        y3 = 0;
    else
        y3 = 1;
    end
else
    y3 = 0;
end

== matlab function rule_DJ/trigger_rule1 ==
  data: Ego input; y_line input; laneEgo input; y1 output; y2 output
function [y1, y2]  = fcn(Ego,y_line,laneEgo)
%%

%参数需求
Egox = Ego.EgoX;                  
Egoy = Ego.EgoY;                  
Egovx = Ego.EgoVx;                
Egovy = Ego.EgoVy;
Egol = Ego.Length;
Egow = Ego.Width;
Egotheta = Ego.EgoTheta;          

if Egovx >0        
    Egotheta = Egotheta;
else
    Egotheta = pi + Egotheta;
end
lf_Ego = Egoy + 0.5 * Egol * sin(Egotheta) - 0.5 * Egow * cos(Egotheta); %左前角车辆横坐标
rf_Ego = Egoy + 0.5 * Egol * sin(Egotheta) + 0.5 * Egow * cos(Egotheta); %右前角车辆横坐标
lr_Ego = Egoy - 0.5 * Egol * sin(Egotheta) - 0.5 * Egow * cos(Egotheta); %左前角车辆横坐标
rr_Ego = Egoy - 0.5 * Egol * sin(Egotheta) + 0.5 * Egow * cos(Egotheta); %右后角车辆横坐标
if Egovx > 0 && Egovy > 0
    changeleft = 1;
    Egoxf_line = polyval(y_line(laneEgo,:),Egox+0.5*Egol*cos(Egotheta));
    changeright = sign((rf_Ego-Egoxf_line) * (lr_Ego-Egoxf_line));
elseif Egovx > 0 && Egovy < 0
    Egoxf_line = polyval(y_line(laneEgo+1,:),Egox+0.5*Egol*cos(Egotheta));
    changeleft = sign((lf_Ego-Egoxf_line) * (rr_Ego-Egoxf_line));
    changeright = 1;
elseif Egovx < 0 && Egovy > 0
    Egoxf_line = polyval(y_line(laneEgo,:),Egox+0.5*Egol*cos(Egotheta));
    changeleft = sign((lf_Ego-Egoxf_line) * (rr_Ego-Egoxf_line));
    changeright = 1;
else
    changeleft = 1;
    Egoxf_line = polyval(y_line(laneEgo+1,:),Egox+0.5*Egol*cos(Egotheta));
    changeright = sign((rf_Ego-Egoxf_line) * (lr_Ego-Egoxf_line));
end

if abs(Egovy)>0.2 && changeleft<=0      %向左换道
    y1 = true;
    y2 = false;
elseif abs(Egovy)>0.2 && changeright<=0     %向右换道
    y1 = false;
    y2 = true;
else
    y1 = false;
    y2 = false;
end

== matlab function rule_DJ/EnabledSubsystem/EnabledSubsystem/distance/beforerchangelane ==
  data: Tgt_f input; Tgt_rf input; Tgt_rr input; y1 output; y2 output; y3 output; Ego input; Threshold_para input
function [y1,y2,y3] = fcn(Tgt_f,Tgt_rf,Tgt_rr,Ego,Threshold_para)
%%参数注释
%{
sEgo = 0;                  %自车纵坐标（始终为零）(m)
dEgo = Ego(2);             %自车横坐标(m)
vxEgo = Ego(3);            %自车纵向速度(m/s)
vyEgo = Ego(4);            %自车横向速度(m/s)
phiEgo = Ego(5);           %自车航向角（相对路径切向夹角，逆时针为正） (rad)
laneEgo = Ego(6);          %自车所在车道
wEgo = Ego(6);             %自车横向宽度(m)
aEgo = Ego(7);             %自车质心到最前端的距离(m)
bEgo = Ego(8);             %自车质心到最前端的距离(m)
sTgt_ot = Tgt_ot(1);         %超车目标纵坐标(m)
dTgt_ot = Tgt_ot(2);         %超车目标横坐标(m)
vxTgt_ot = Tgt_ot(3);        %超车目标纵向速度(m/s)
vyTgt_ot = Tgt_ot(4);        %超车目标横向速度(m/s)
sTgt_f = Tgt_f(1);         %前车纵坐标(m)
dTgt_f = Tgt_f(2);         %前车横坐标(m)
vxTgt_f = Tgt_f(3);        %前车纵向速度(m/s)
vyTgt_f = Tgt_f(4);        %前车横向速度(m/s)
sTgt_lf = Tgt_lf(1);       %左前车纵坐标(m)
dTgt_lf = Tgt_lf(2);       %左前车横坐标(m)
vxTgt_lf = Tgt_lf(3);      %左前车纵向速度(m/s)
vyTgt_lf = Tgt_lf(4);      %左前车横向速度(m/s)
Tgt_lr, Tgt_rf, Tgt_rr与左前车类似，分别表示相对自车的左后车辆，右前车辆以及右后车辆
dlaneline =[dlaneline-1,dlaneline-2,……]
%同向车道内车道线横向坐标集，最靠近道路中心线的一侧为-1，往外依次递减
TTCx_f = Threshold_para(1);             %纵向安全距离
TTCx_lr = Threshold_para(2);            %超车道后方安全距离
TTCx_lf = Threshold_para(3);            %超车道前方安全距离
t_chngln = Threshold_para(4);           %换道持续最大时间
overtake_deltav = Threshold_para(5);    %超车速度差
sf_dist_return = Threshold_para(6);     %返回原车道与后方车辆的安全，由于超车时自车速度应大于被超车辆
TTCx_rf = Threshold_para(7);            %原车道前方安全距离
%}
%%

%参数需求

Tgtx_rr = Tgt_rr(1);              %frenet坐标系下左侧车道后方车辆坐标
Tgty_rr = Tgt_rr(2);              
Egox = Ego.EgoX;                    %自车纵坐标（）
Egovx = Ego.EgoVx;                  %自车纵向速度(m/s)
Tgtx_f = Tgt_f(1);              %超车目标纵坐标(m)
Tgty_f = Tgt_f(2);
Tgtvx_f = Tgt_f(3);             %超车目标纵向速度(m/s)
Tgtx_rf = Tgt_rf(1);              %frenet坐标系下左侧车道前方车辆坐标
Tgty_rf = Tgt_rf(2);
Tgtvx_rf = Tgt_rf(3);             %左前车纵向速度(m/s)
TTCx = Threshold_para(7);      %安全碰撞时间

%与前车的安全距离判断
if Tgtx_f ~= 2000 && Tgty_f ~= 2000 && abs(Egovx)>abs(Tgtvx_f)    %坐标不为0视为存在左前车
    if abs(Tgtx_f-Egox) >= abs(Egovx - Tgtvx_f) * TTCx 
        y1 = 0;
    else
        y1 = 1;
    end
else
    y1 = 0;
end
%与右前车的安全距离判断
if Tgtx_rf ~= 2000 && Tgty_rf ~= 2000 && abs(Egovx)>abs(Tgtvx_rf)    %坐标不为0视为存在左前车
    if abs(Tgtx_rf-Egox) >= abs(Egovx - Tgtvx_rf) * TTCx 
        y2 = 0;
    else
        y2 = 1;
    end
else
    y2 = 0;
end
%与左后车的安全距离判断
if Tgtx_rr ~= 2000 && Tgty_rr ~= 2000     %坐标不为0视为存在左后车
    if abs(Tgtx_rr-Egox) >= 10
        y3 = 0;
    else
        y3 = 1;
    end
else
    y3 = 0;
end

== matlab function rule_DJ/change_left/beforeovertaking ==
  data: y1 output; y2 output; y3 output; Ego input; Tgt_f input; Tgt_lf input; Tgt_lr input; Threshold_para input; Y1 output; Y2 output; Y3 output
function [y1,y2,y3,Y1,Y2,Y3] = fcn(Ego,Tgt_f,Tgt_lf,Tgt_lr,Threshold_para)
%%

%参数需求

Tgtx_lr = Tgt_lr(1);              
Tgty_lr = Tgt_lr(2);              
Tgtvx_lr = Tgt_lr(3);             
Tgtl_lr = Tgt_lr(4);
Egox = Ego.EgoX;                    
Egovx = Ego.EgoVx;                  
Egol = Ego.Length;
Tgtx_f = Tgt_f(1);              
Tgty_f = Tgt_f(2);
Tgtvx_f = Tgt_f(3);             
Tgtl_f = Tgt_f(4);
Tgtx_lf = Tgt_lf(1);              
Tgty_lf = Tgt_lf(2);
Tgtl_lf = Tgt_lf(4);
Tgtvx_lf = Tgt_lf(3);             
TTCx = Threshold_para(7);      
dclmin = Threshold_para(9);

%与前车的安全距离判断
if Tgtx_f ~= 2000 && Tgty_f ~= 2000 && abs(Egovx)>abs(Tgtvx_f)    %坐标不为0视为存在前车
    if abs(Tgtx_f-Egox) >= abs(Egovx - Tgtvx_f) * TTCx || abs(Tgtx_f-Egox) -0.5*(Tgtl_f+Egol) >= dclmin
        y1 = 0;
    else
        y1 = 1;
    end
    Y1 = abs(Tgtx_f-Egox) -0.5*(Tgtl_f+Egol);
else
    y1 = 0;
    Y1 = 2000;
end

%与左前车的安全距离判断
if Tgtx_lf ~= 2000 && Tgty_lf ~= 2000 && abs(Egovx)>abs(Tgtvx_lf)    %坐标不为0视为存在左前车
    if abs(Tgtx_lf-Egox) >= abs(Egovx - Tgtvx_lf) * TTCx || abs(Tgtx_lf-Egox) -0.5*(Tgtl_lf+Egol) >= dclmin
        y2 = 0;
    else
        y2 = 1;
    end
    Y2 = abs(Tgtx_lf-Egox) -0.5*(Tgtl_lf+Egol);
else
    y2 = 0;
    Y2 = 2000;
end

%与左后车的安全距离判断
if Tgtx_lr ~= 2000 && Tgty_lr ~= 2000 && abs(Egovx)<abs(Tgtvx_lr)    %坐标不为0视为存在左后车
    if abs(Tgtx_lr-Egox) >= abs(Egovx - Tgtvx_lr) * TTCx || abs(Tgtx_lr-Egox) -0.5*(Tgtl_lr+Egol) >= dclmin
        y3 = 0;
    else
        y3 = 1;
    end
    Y3 = abs(Tgtx_lr-Egox) -0.5*(Tgtl_lr+Egol);
else
    y3 = 0;
    Y3 = 2000;
end

== matlab function rule_DJ/trigger_rule80 ==
  data: y output; Egolaneid input; y_line input
function y = fcn(Egolaneid,y_line)
%%

%参数需求
lane_type = Egolaneid;

%高速主路限速触发条件判断
if lane_type ~= 1 && lane_type ~= size(y_line,1)-1        %自车所属车道类型为主干道则条件有效
    y = 1;
else
    y = 0;
end

== matlab function rule_DJ/rule80/高速保持车距监测 ==
  data: y output; Ego input; Tgt_f input; y2 output; Cd output
function [y,y2,Cd] = fcn(Ego,Tgt_f)
%%
%参数需求
Tgtx_f = Tgt_f(1);              %目标纵坐标(m)
Tgty_f = Tgt_f(2);              %目标横坐标(m)
Tgtl_f = Tgt_f(4);              %目标长度(m)
Egox = Ego.EgoX;                %自车纵坐标（0）
Egovx = Ego.EgoVx;              %自车纵向速度(m/s)
Egol = Ego.Length;              %自车长度(m)

if Tgtx_f ~=2000 && Tgty_f ~=2000     %坐标不为0视为存在前车
    if abs(Egovx) >= 100/3.6
        Cd = 100;
        if abs(Tgtx_f-Egox)-0.5*(Tgtl_f+Egol) >100
            y = 0;
        else
            y = 1;
        end
    else
        Cd =50;
        if abs(Tgtx_f-Egox)-0.5*(Tgtl_f+Egol) >50
            y = 0;
        else
            y = 1;
        end
    end
    y2 = abs(Tgtx_f-Egox)-0.5*(Tgtl_f+Egol);
else
    y = 0;
    y2 = 2000;
    Cd = 0;
end

== matlab function rule_DJ/change_left/zoning ==
  data: Ego input; Tgt_f output; Tgt input; y_line input; Tgt_b output; Tgt_lf output; Tgt_lr output; Tgt_rf output; Tgt_rr output; Egolane output
function [Tgt_f,Tgt_b,Tgt_lf,Tgt_lr,Tgt_rf,Tgt_rr,Egolane] = fcn(Ego,Tgt,y_line)
%{
根据HighD数据集提供的信息，通过确定自车所在的位置，以及他车的坐标，判断他车相对于自车的方位
%}
Egox = Ego.EgoX;
Egoy = Ego.EgoY;
Egovx = Ego.EgoVx;
Tgtx = Tgt.TgtX;
Tgty = Tgt.TgtY;
Tgtvx = Tgt.TgtVx;
Tgtl = Tgt.Length;
Tgtw = Tgt.Width;

%%判断自车所在的车道
for i = 1:size(y_line,1)
    if Egoy >= polyval(y_line(i,:),Egox);
        Egolane = i-1;
        break
    else
        Egolane = i;
    end
end

%%对周围的他车进行方位分割
if Egolane<size(y_line,1)/2  %说明自车在地图中为向右行驶（下方）车辆
    Flag1 = Tgtx > Egox;      %他车位于自车之前
    Flag2 = Tgtx <= Egox;     %他车位于自车之后
    if Egolane == 1                                   %自车位于车道1
        Flag3 = (Tgty>=polyval(y_line(2,:),Tgtx) & Tgty<polyval(y_line(1,:),Tgtx));      %同车道他车
        Flag5 = (Tgty>=polyval(y_line(3,:),Tgtx) & Tgty<polyval(y_line(2,:),Tgtx));;      %左侧车道他车
        [m, n] = size(Flag3);
        Flag4 = false(m,n);%右侧车道他车
    elseif Egolane>1 && Egolane<size(y_line,1)/2           %自车位于车道中间车道
        Flag3 = (Tgty>=polyval(y_line(Egolane+1,:),Tgtx) & Tgty<polyval(y_line(Egolane,:),Tgtx));   %同车道他车
        Flag5 = (Tgty>=polyval(y_line(Egolane+2,:),Tgtx) & Tgty<polyval(y_line(Egolane+1,:),Tgtx)); %左侧车道他车
        Flag4 = (Tgty>=polyval(y_line(Egolane,:),Tgtx) & Tgty<polyval(y_line(Egolane-1,:),Tgtx));   %右侧车道他车
    else                                                  %自车位于车道3
        Flag3 = (Tgty>=polyval(y_line(Egolane+1,:),Tgtx) & Tgty<polyval(y_line(Egolane,:),Tgtx));  %同车道他车
        [m, n] = size(Flag3);
        Flag5 = false(m,n);
        Flag4 = (Tgty>=polyval(y_line(Egolane,:),Tgtx) & Tgty<polyval(y_line(Egolane-1,:),Tgtx));  %右侧车道他车
    end
else
    Flag1 = Tgtx <= Egox;    %他车位于自车之前
    Flag2 = Tgtx > Egox;     %他车位于自车之后
    if Egolane == size(y_line,1)/2+1                                   %自车位于车道6
        Flag3 = (Tgty>=polyval(y_line(Egolane+1,:),Tgtx) & Tgty<polyval(y_line(Egolane,:),Tgtx));  %同车道他车
        Flag4 = (Tgty>=polyval(y_line(Egolane+2,:),Tgtx) & Tgty<polyval(y_line(Egolane+1,:),Tgtx));  %右侧车道他车
        [m, n] = size(Flag3);
        Flag5 = false(m,n);
    elseif Egolane>size(y_line,1)/2+1 && Egolane<=size(y_line,1)-2           %自车位于车道-2
        Flag3 = (Tgty>=polyval(y_line(Egolane+1,:),Tgtx) & Tgty<polyval(y_line(Egolane,:),Tgtx));  %同车道他车
        Flag4 = (Tgty>=polyval(y_line(Egolane+2,:),Tgtx) & Tgty<polyval(y_line(Egolane+1,:),Tgtx));  %右侧车道他车
        Flag5 = (Tgty>=polyval(y_line(Egolane,:),Tgtx) & Tgty<polyval(y_line(Egolane-1,:),Tgtx));  %左侧车道他车
    else                                                  %自车位于车道-3
        Flag3 = (Tgty>=polyval(y_line(Egolane+1,:),Tgtx) & Tgty<polyval(y_line(Egolane,:),Tgtx));               %同车道他车
        [m, n] = size(Flag3);
        Flag4 = false(m,n);
        Flag5 = (Tgty>=polyval(y_line(Egolane,:),Tgtx) & Tgty<polyval(y_line(Egolane+1,:),Tgtx)); %左侧车道他车
    end
end

%%筛选六个方位中离自车最近的车，即每个方位区域只保留一辆车
Flag_f = Flag1 & Flag3;      %同车道前车
if any(Flag_f)
    f_min = min(abs(Tgtx(Flag_f) - Egox));
    Tgtx_f = (sign(min(Tgtx(Flag_f) - Egox)) * f_min) + Egox;
    [col_f,~] = find(abs(Tgtx-Tgtx_f)<=0.0001 & Flag_f == true);
    if ~isempty(col_f)
        Tgty_f = Tgty(col_f(1));
        Tgtvx_f = Tgtvx(col_f(1));
        Tgtl_f = Tgtl(col_f(1));
        Tgtw_f = Tgtw(col_f(1));
    else
        Tgty_f = 0;
        Tgtvx_f = 0;
        Tgtl_f = 0;
        Tgtw_f = 0;
    end
else
    f_min = 0;
    Tgtx_f = 2000;
    Tgty_f = 2000;
    Tgtvx_f = 2000;
    Tgtl_f = 2000;
    Tgtw_f = 2000;
end
Tgt_f = [Tgtx_f, Tgty_f, Tgtvx_f, Tgtl_f, Tgtw_f];
Flag_b = Flag2 & Flag3;      %同车道后车
if any(Flag_b)
    b_min = min(abs(Tgtx(Flag_b) - Egox));
    Tgtx_b = (sign(min(Tgtx(Flag_b) - Egox)) * b_min) + Egox;
    [col_b,~] = find(abs(Tgtx-Tgtx_b)<=0.0001 & Flag_b == true);
    if ~isempty(col_b)
        Tgty_b = Tgty(col_b(1));
        Tgtvx_b = Tgtvx(col_b(1));
        Tgtl_b = Tgtl(col_b(1));
        Tgtw_b = Tgtw(col_b(1));
    else
        Tgty_b = 0;
        Tgtvx_b = 0;
        Tgtl_b = 0;
        Tgtw_b = 0;
    end
else
    b_min = 0;
    Tgtx_b = 2000;
    Tgty_b = 2000;
    Tgtvx_b = 2000;
    Tgtl_b = 2000;
    Tgtw_b = 2000;
end
Tgt_b = [Tgtx_b, Tgty_b, Tgtvx_b, Tgtl_b, Tgtw_b];
Flag_lf = (Flag1 & Flag5);     %左侧车道前车
if any(Flag_lf)
    lf_min = min(abs(Tgtx(Flag_lf) - Egox));
    Tgtx_lf = (sign(min(Tgtx(Flag_lf) - Egox)) * lf_min) + Egox;
    [col_lf,~] = find(abs(Tgtx-Tgtx_lf)<=0.0001 & Flag_lf == true);
    if ~isempty(col_lf)
        Tgty_lf = Tgty(col_lf(1));
        Tgtvx_lf = Tgtvx(col_lf(1));
        Tgtl_lf = Tgtl(col_lf(1));
        Tgtw_lf = Tgtw(col_lf(1));
    else
        Tgty_lf = 0;
        Tgtvx_lf = 0;
        Tgtl_lf = 0;
        Tgtw_lf = 0;
    end
else
    lf_min = 0;
    Tgtx_lf = 2000;
    Tgty_lf = 2000;
    Tgtvx_lf = 2000;
    Tgtl_lf = 2000;
    Tgtw_lf = 2000;
end
Tgt_lf = [Tgtx_lf, Tgty_lf, Tgtvx_lf, Tgtl_lf, Tgtw_lf];
Flag_lr = Flag2 & Flag5;     %左侧车道后车
if any(Flag_lr)
    lr_min = min(abs(Tgtx(Flag_lr) - Egox));
    Tgtx_lr = (sign(min(Tgtx(Flag_lr) - Egox)) * lr_min) + Egox;
    [col_lr,~] = find(abs(Tgtx-Tgtx_lr)<=0.0001 & Flag_lr == true);
    if ~isempty(col_lr)
        Tgty_lr = Tgty(col_lr(1));
        Tgtvx_lr = Tgtvx(col_lr(1));
        Tgtl_lr = Tgtl(col_lr(1));
        Tgtw_lr = Tgtw(col_lr(1));
    else
        Tgty_lr = 0;
        Tgtvx_lr = 0;
        Tgtl_lr = 0;
        Tgtw_lr = 0;
    end
else
    lr_min = 0;
    Tgtx_lr= 2000;
    Tgty_lr = 2000;
    Tgtvx_lr = 2000;
    Tgtl_lr = 2000;
    Tgtw_lr = 2000;
end
Tgt_lr = [Tgtx_lr, Tgty_lr, Tgtvx_lr, Tgtl_lr, Tgtw_lr];
Flag_rf = Flag1 & Flag4;     %右侧车道前车
if any(Flag_rf)
    rf_min = min(abs(Tgtx(Flag_rf) - Egox));
    Tgtx_rf = (sign(min(Tgtx(Flag_rf) - Egox)) * rf_min) + Egox;
    [col_rf,~] = find(abs(Tgtx-Tgtx_rf)<=0.0001 & Flag_rf == true);
    if ~isempty(col_rf)
        Tgty_rf = Tgty(col_rf(1));
        Tgtvx_rf = Tgtvx(col_rf(1));
        Tgtl_rf = Tgtl(col_rf(1));
        Tgtw_rf = Tgtw(col_rf(1));
    else
        Tgty_rf = 0;
        Tgtvx_rf = 0;
        Tgtl_rf = 0;
        Tgtw_rf = 0;
    end
else
    rf_min = 0;
    Tgtx_rf = 2000;
    Tgty_rf = 2000;
    Tgtvx_rf = 2000;
    Tgtl_rf = 2000;
    Tgtw_rf = 2000;
end
Tgt_rf = [Tgtx_rf, Tgty_rf, Tgtvx_rf, Tgtl_rf, Tgtw_rf];
Flag_rr = Flag2 & Flag4;     %同车道后车
if any(Flag_rr)
    rr_min = min(abs(Tgtx(Flag_rr) - Egox));
    Tgtx_rr = (sign(min(Tgtx(Flag_rr) - Egox)) * rr_min) + Egox;
    [col_rr,~] = find(abs(Tgtx-Tgtx_rr)<=0.0001 & Flag_rr == true);
    if ~isempty(col_rr)
        Tgty_rr = Tgty(col_rr(1));
        Tgtvx_rr = Tgtvx(col_rr(1));
        Tgtl_rr = Tgtl(col_rr(1));
        Tgtw_rr = Tgtw(col_rr(1));
    else
        Tgty_rr = 0;
        Tgtvx_rr = 0;
        Tgtl_rr = 0;
        Tgtw_rr = 0;
    end
else
    rr_min = 0;
    Tgtx_rr = 2000;
    Tgty_rr = 2000;
    Tgtvx_rr = 2000;
    Tgtl_rr = 2000;
    Tgtw_rr = 2000;
end
Tgt_rr = [Tgtx_rr, Tgty_rr, Tgtvx_rr, Tgtl_rr, Tgtw_rr];

== matlab function rule_DJ/change_right/beforerchangelane ==
  data: Tgt_f input; Tgt_rf input; Tgt_rr input; y1 output; y2 output; y3 output; Ego input; Threshold_para input; Y1 output; Y2 output; Y3 output
function [y1,y2,y3,Y1,Y2,Y3] = fcn(Tgt_f,Tgt_rf,Tgt_rr,Ego,Threshold_para)
%%

%参数需求

Tgtx_rr = Tgt_rr(1);             
Tgty_rr = Tgt_rr(2);              
Tgtvx_rr = Tgt_rr(3);
Tgtl_rr = Tgt_rr(4);
Egox = Ego.EgoX;                    %自车纵坐标（）
Egovx = Ego.EgoVx;                  %自车纵向速度(m/s)
Egol = Ego.Length;
Tgtx_f = Tgt_f(1);              
Tgty_f = Tgt_f(2);
Tgtvx_f = Tgt_f(3);            
Tgtl_f = Tgt_f(4);
Tgtx_rf = Tgt_rf(1);              
Tgty_rf = Tgt_rf(2);
Tgtvx_rf = Tgt_rf(3);            
Tgtl_rf = Tgt_rf(4);            
TTCx = Threshold_para(7);      %安全碰撞时间
dclmin = Threshold_para(9);      %换道最低距离

%与前车的安全距离判断
if Tgtx_f ~= 2000 && Tgty_f ~= 2000 && abs(Egovx)>abs(Tgtvx_f)     %坐标不为0视为存在前车
    if abs(Tgtx_f-Egox) >= abs(Egovx - Tgtvx_f) * TTCx || abs(Tgtx_f-Egox)-0.5*(Tgtl_f+Egol) >= dclmin
        y1 = 0;
    else
        y1 = 1;
    end
    Y1 = abs(Tgtx_f-Egox)-0.5*(Tgtl_f+Egol);
else
    y1 = 0;
    Y1 = 2000;
end
%与右前车的安全距离判断
if Tgtx_rf ~= 2000 && Tgty_rf ~= 2000 && abs(Egovx)>abs(Tgtvx_rf)    %坐标不为0视为存在右前车
    if abs(Tgtx_rf-Egox) >= abs(Egovx - Tgtvx_rf) * TTCx || abs(Tgtx_rf-Egox)-0.5*(Tgtl_rf+Egol) >= dclmin
        y2 = 0;
    else
        y2 = 1;
    end
    Y2 = max(abs(Tgtx_rf-Egox)-0.5*(Tgtl_rf+Egol),0);
else
    y2 = 0;
    Y2 = 2000;
end
%与右后车的安全距离判断
if Tgtx_rr ~= 2000 && Tgty_rr ~= 2000 && abs(Egovx)<abs(Tgtvx_rr)    %坐标不为0视为存在右后车
    if abs(Tgtx_rr-Egox) >= abs(Egovx - Tgtvx_rr) * TTCx || abs(Tgtx_rr-Egox)-0.5*(Tgtl_rr+Egol) >= dclmin
        y3 = 0;
    else
        y3 = 1;
    end
    Y3 = max(abs(Tgtx_rr-Egox)-0.5*(Tgtl_rr+Egol),0);
else
    y3 = 0;
    Y3 = 2000;
end

== matlab function rule_DJ/EnabledSubsystem/EnabledSubsystem1/changeright ==
  data: Egolane input; initial_lane input; Ego input; y_line input; cmplt_change output
function cmplt_change  = fcn(Egolane,initial_lane,Ego,y_line)
%%参数注释
%{
sEgo = 0;                  %自车纵坐标（始终为零）(m)
dEgo = Ego(2);             %自车横坐标(m)
vxEgo = Ego(3);            %自车纵向速度(m/s)
vyEgo = Ego(4);            %自车横向速度(m/s)
phiEgo = Ego(5);           %自车航向角（相对路径切向夹角，逆时针为正） (rad)
laneEgo = Ego(6);          %自车所在车道
wEgo = Ego(7);             %自车横向宽度(m)
aEgo = Ego(8);             %自车质心到最前端的距离(m)
bEgo = Ego(9);             %自车质心到最前端的距离(m)
sTgt_ot = Tgt_ot(1);       %超车目标纵坐标(m)
dTgt_ot = Tgt_ot(2);       %超车目标横坐标(m)
vxTgt_ot = Tgt_ot(3);      %超车目标纵向速度(m/s)
vyTgt_ot = Tgt_ot(4);      %超车目标横向速度(m/s)
sTgt_f = Tgt_f(1);         %前车纵坐标(m)
dTgt_f = Tgt_f(2);         %前车横坐标(m)
vxTgt_f = Tgt_f(3);        %前车纵向速度(m/s)
vyTgt_f = Tgt_f(4);        %前车横向速度(m/s)
sTgt_lf = Tgt_lf(1);       %左前车纵坐标(m)
dTgt_lf = Tgt_lf(2);       %左前车横坐标(m)
vxTgt_lf = Tgt_lf(3);      %左前车纵向速度(m/s)
vyTgt_lf = Tgt_lf(4);      %左前车横向速度(m/s)
Tgt_lr, Tgt_rf, Tgt_rr与左前车类似，分别表示相对自车的左后车辆，右前车辆以及右后车辆
dlaneline =[dlaneline-1,dlaneline-2,……]
%同向车道内车道线横向坐标集，最靠近道路中心线的一侧为-1，往外依次递减
TTCx_f = Threshold_para(1);             %纵向安全距离
TTCx_lr = Threshold_para(2);            %超车道后方安全距离
TTCx_lf = Threshold_para(3);            %超车道前方安全距离
t_chngln = Threshold_para(4);           %换道持续最大时间
overtake_deltav = Threshold_para(5);    %超车速度差
sf_dist_return = Threshold_para(6);     %返回原车道与后方车辆的安全，由于超车时自车速度应大于被超车辆
TTCx_rf = Threshold_para(7);            %原车道前方安全距离
%}
%%

%参数需求
Egox = Ego.EgoX; 
Egoy = Ego.EgoY;                    %自车y坐标(m)
Egovx = Ego.EgoVx;
Egovy = Ego.EgoVy;
Egol = Ego.Length;
Egow = Ego.Width;
Egotheta = Ego.EgoTheta;
laneEgo = Egolane;          %自车所在车道


%计算向左换道所用时间
lf_Ego = Egoy + 0.5 * Egol * sin(Egotheta) - 0.5 * Egow * cos(Egotheta); %左前角车辆横坐标
rf_Ego = Egoy + 0.5 * Egol * sin(Egotheta) + 0.5 * Egow * cos(Egotheta); %右前角车辆横坐标
lr_Ego = Egoy - 0.5 * Egol * sin(Egotheta) - 0.5 * Egow * cos(Egotheta); %左前角车辆横坐标
rr_Ego = Egoy - 0.5 * Egol * sin(Egotheta) + 0.5 * Egow * cos(Egotheta); %右后角车辆横坐标

if Egovx > 0 && Egovy > 0
    changeleft = 1;
    Egoxf_line = polyval(y_line(initial_lane,:),Egox+0.5*Egol*cos(Egotheta));
    changeright = sign((rf_Ego-Egoxf_line) * (lr_Ego-Egoxf_line));
elseif Egovx > 0 && Egovy < 0
    Egoxf_line = polyval(y_line(initial_lane+1,:),Egox+0.5*Egol*cos(Egotheta));
    changeleft = sign((lf_Ego-Egoxf_line) * (rr_Ego-Egoxf_line));
    changeright = 1;
elseif Egovx < 0 && Egovy > 0
    Egoxf_line = polyval(y_line(initial_lane,:),Egox+0.5*Egol*cos(Egotheta));
    changeleft = sign((lf_Ego-Egoxf_line) * (rr_Ego-Egoxf_line));
    changeright = 1;
else
    changeleft = 1;
    Egoxf_line = polyval(y_line(initial_lane+1,:),Egox+0.5*Egol*cos(Egotheta));
    changeright = sign((rf_Ego-Egoxf_line) * (lr_Ego-Egoxf_line));
end

if Egovx > 0
    if laneEgo == initial_lane && changeleft > 0 && changeright > 0
        cmplt_change = 1;
    elseif laneEgo == initial_lane-1 && changeleft > 0 && changeright > 0
        cmplt_change = 2;
    elseif laneEgo == initial_lane-1 && changeleft <= 0
        cmplt_change = 4;
    else 
        cmplt_change = 0;
    end
else
    if laneEgo == initial_lane && changeleft > 0 && changeright > 0
        cmplt_change = 1;
    elseif laneEgo == initial_lane+1 && changeleft > 0 && changeright > 0
        cmplt_change = 2;
    elseif laneEgo == initial_lane+1 && changeleft <= 0
        cmplt_change = 4;
    else 
        cmplt_change = 0;
    end
end

end

== matlab function rule_DJ/EnabledSubsystem/EnabledSubsystem1/distance/beforerchangelane ==
  data: Tgt_lr input; y3 output; Ego input; Threshold_para input
function y3  = fcn(Tgt_lr,Ego,Threshold_para)
%%参数注释
%{
sEgo = 0;                  %自车纵坐标（始终为零）(m)
dEgo = Ego(2);             %自车横坐标(m)
vxEgo = Ego(3);            %自车纵向速度(m/s)
vyEgo = Ego(4);            %自车横向速度(m/s)
phiEgo = Ego(5);           %自车航向角（相对路径切向夹角，逆时针为正） (rad)
laneEgo = Ego(6);          %自车所在车道
wEgo = Ego(6);             %自车横向宽度(m)
aEgo = Ego(7);             %自车质心到最前端的距离(m)
bEgo = Ego(8);             %自车质心到最前端的距离(m)
sTgt_ot = Tgt_ot(1);         %超车目标纵坐标(m)
dTgt_ot = Tgt_ot(2);         %超车目标横坐标(m)
vxTgt_ot = Tgt_ot(3);        %超车目标纵向速度(m/s)
vyTgt_ot = Tgt_ot(4);        %超车目标横向速度(m/s)
sTgt_f = Tgt_f(1);         %前车纵坐标(m)
dTgt_f = Tgt_f(2);         %前车横坐标(m)
vxTgt_f = Tgt_f(3);        %前车纵向速度(m/s)
vyTgt_f = Tgt_f(4);        %前车横向速度(m/s)
sTgt_lf = Tgt_lf(1);       %左前车纵坐标(m)
dTgt_lf = Tgt_lf(2);       %左前车横坐标(m)
vxTgt_lf = Tgt_lf(3);      %左前车纵向速度(m/s)
vyTgt_lf = Tgt_lf(4);      %左前车横向速度(m/s)
Tgt_lr, Tgt_rf, Tgt_rr与左前车类似，分别表示相对自车的左后车辆，右前车辆以及右后车辆
dlaneline =[dlaneline-1,dlaneline-2,……]
%同向车道内车道线横向坐标集，最靠近道路中心线的一侧为-1，往外依次递减
TTCx_f = Threshold_para(1);             %纵向安全距离
TTCx_lr = Threshold_para(2);            %超车道后方安全距离
TTCx_lf = Threshold_para(3);            %超车道前方安全距离
t_chngln = Threshold_para(4);           %换道持续最大时间
overtake_deltav = Threshold_para(5);    %超车速度差
sf_dist_return = Threshold_para(6);     %返回原车道与后方车辆的安全，由于超车时自车速度应大于被超车辆
TTCx_rf = Threshold_para(7);            %原车道前方安全距离
%}
%%

%参数需求
Tgtx_lr = Tgt_lr(1);
Tgty_lr = Tgt_lr(2);
Tgtvx_lr = Tgt_lr(3);
Egox = Ego.EgoX;                    %自车纵坐标（）
Egovx = Ego.EgoVx;                  %自车纵向速度(m/s)
TTCx = Threshold_para(7);      %安全碰撞时间

%与左后车的安全距离判断
if Tgtx_lr ~= 2000 && Tgty_lr ~=2000     %坐标不为2000视为存在左后车
    if abs(Tgtx_lr-Egox) <= abs(Egovx - Tgtvx_lr) * TTCx || ...,
            abs(Tgtx_lr-Egox) <= 20
        y3 = 1;
    else
        y3 = 0;
    end
else
    y3 = 0;
end
